simulink model "lead_acid_bat_eq_ckt_CC"  (R2025b)
settings: Solver=VariableStepAuto  StartTime=0.0  StopTime=200  RelTol=1e-3
libraries: fl_lib x16, nesl_utility x9, ee_lib x2
settings Model: Creator=huhry  LastModifiedBy=Hari
settings DebuggingCC: AlgebraicLoopMsg=none

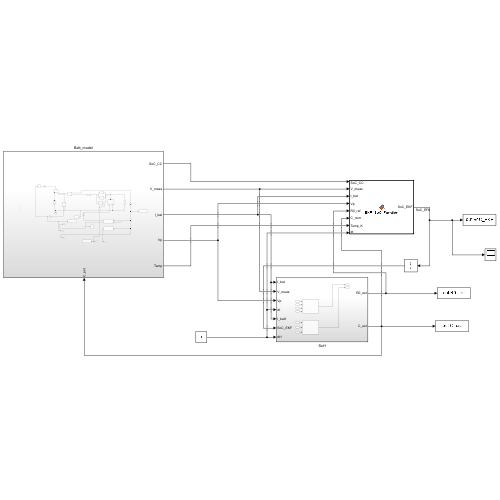
[thumbnail: Simulink's stored preview of the top-level diagram]
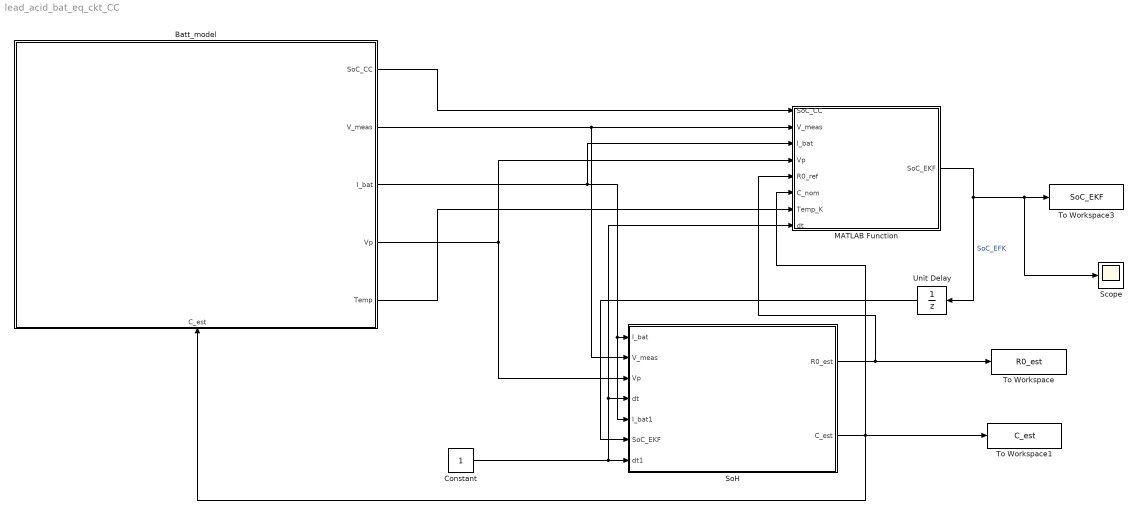
== system lead_acid_bat_eq_ckt_CC ==
  Batt_model : Subsystem
      settings: PortSchema="{\"entries\":[{\"content\":{\"sides\":[{\"content\":{},\"type\":\"ConnectorPlacement.EquallySpacedRectSide\",\"uuid\":\"49c69b95-09c6-49fd-b891-4f09856a00b3\"},{\"content\":{\"connectorIds\":[\"Out1\",\"Out2\",\"Out3\",\"Out4\",\"Out5\"],\"side\":\"RIGHT\"},\"type\":\"ConnectorPlacement.EquallySpacedRectSide\",\"uuid\":\"811e1f4c-4865-4a20-acff-08171fe05a53\"},{\"content\":{\"side\":\"TOP\"},\"type\":\"ConnectorPlacement.EquallySpacedRectSide\",\"uuid\":\"82a5ceef-4616-42bd-9951-d3b757a6a369\"},{\"content\":{\"connectorIds\":[\"In1\"],\"side\":\"BOTTOM\"},\"type\":\"ConnectorPlacement.EquallySpacedRectSide\",\"uuid\":\"0331ad85-3468-4588-880b-20861dbd2507\"}]},\"type\":\"ConnectorPlacement.EquallySpacedConnector\",\"uuid\":\"59096161-8cd8-4eb0-902d-7fdbb6e4005d\"}],\"packageUris\":[\"http://schema.mathworks.com/mf0/Connector/R2020b\"],\"version\":\"1.0\"}"
  Constant : Constant
  MATLAB Function : MATLAB Function  TreatAsAtomicUnit=on  SystemSampleTime=1
  Scope : Scope
      settings: ActiveDisplayYMinimum=-0.0893057108045884  ActiveDisplayYMaximum=1.1210339678671766
  SoH : Subsystem
  To Workspace : ToWorkspace  VariableName=R0_est  SaveFormat=Timeseries  SampleTime=-1
  To Workspace1 : ToWorkspace  VariableName=C_est  SaveFormat=Timeseries  SampleTime=-1
  To Workspace3 : ToWorkspace  VariableName=SoC_EKF  SaveFormat=Timeseries  SampleTime=-1
  Unit Delay : UnitDelay  InitialCondition=0.1  HasFrameUpgradeWarning=on
  wires:
  MATLAB Function/1(SoC_EKF) -> Unit Delay/1, Scope/1, To Workspace3/1  "SoC_EFK"
  Batt_model/1(SoC_CC) -> MATLAB Function/1(SoC_CC)
  Batt_model/2(V_meas) -> SoH/2(V_meas), MATLAB Function/2(V_meas)
  Batt_model/3(I_bat) -> SoH/5(I_bat1), SoH/1(I_bat), MATLAB Function/3(I_bat)
  Batt_model/4(Vp) -> SoH/3(Vp), MATLAB Function/4(Vp)
  Batt_model/5(Temp) -> MATLAB Function/7(Temp_K)
  SoH/1(R0_est) -> To Workspace/1, MATLAB Function/5(R0_ref)
  Constant/1 -> MATLAB Function/8(dt), SoH/4(dt), SoH/7(dt1)
  Unit Delay/1 -> SoH/6(SoC_EKF)
  SoH/2(C_est) -> Batt_model/1(C_est), To Workspace1/1, MATLAB Function/6(C_nom)

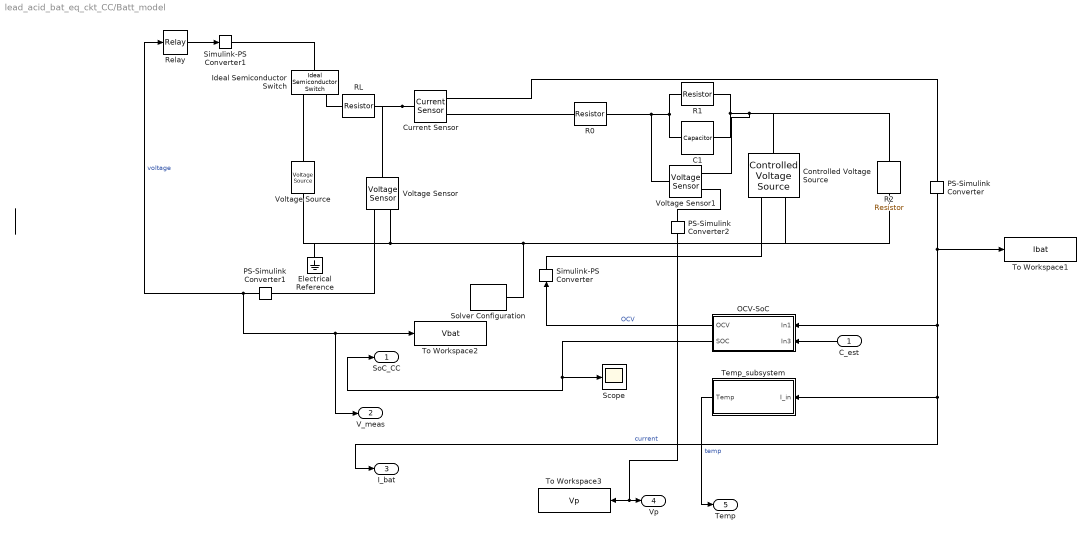
== system lead_acid_bat_eq_ckt_CC/Batt_model ==
  C_est : Inport
  C1 : fl_lib/Electrical/Electrical Elements/Capacitor  c=1000 F  r=1e-6 Ohm  g=0 1/Ohm  i_specify=off  i_priority=None  i=0 A  i_nominal_specify=off  i_nominal_value=1  i_nominal_unit=A  v_specify=off  v_priority=None  v=0 V  v_nominal_specify=off  v_nominal_value=1  v_nominal_unit=V  vc_specify=off  vc_priority=High  vc=0 V  vc_nominal_specify=off  vc_nominal_value=1  vc_nominal_unit=V
  Controlled Voltage Source : fl_lib/Electrical/Electrical Sources/Controlled Voltage Source
  Current Sensor : fl_lib/Electrical/Electrical Sensors/Current Sensor
  Electrical Reference : fl_lib/Electrical/Electrical Elements/Electrical Reference
  Ideal Semiconductor Switch : ee_lib/Semiconductors & Converters/Ideal Semiconductor Switch  port_option=ee.enum.controlport.ps  Ron=0.001 Ohm  Goff=1e-6 1/Ohm  Vth=0.5 V  diode_param=ee.enum.semiconductors.protectionDiode.external  diode_Vf=0.8 V  diode_Ron=0.001 Ohm  diode_Goff=1e-5 1/Ohm  diode_C=50e-9 F  diode_iRM=-235 A  diode_iF=300 A  diode_idot=-50 A/us  diode_trr_param=ee.enum.converters.diodetrr.trr_factor  diode_trr_factor=3  diode_trr=15 us  diode_Qrr=1500 s*uA
  OCV-SoC : Subsystem
  PS-Simulink Converter : nesl_utility/PS-Simulink Converter  PhysicalDomain=network_engine_domain  SubClassName=ps_output  LeftPortType=input  RightPortType=output  PseudoPeriodic=off  Frequencies=[]  VectorFormat=inherit  Unit=inherit  AffineConversion=off
  PS-Simulink Converter1 : nesl_utility/PS-Simulink Converter  PhysicalDomain=network_engine_domain  SubClassName=ps_output  LeftPortType=input  RightPortType=output  PseudoPeriodic=off  Frequencies=[]  VectorFormat=inherit  Unit=inherit  AffineConversion=off
  PS-Simulink Converter2 : nesl_utility/PS-Simulink Converter  PhysicalDomain=network_engine_domain  SubClassName=ps_output  LeftPortType=input  RightPortType=output  PseudoPeriodic=off  Frequencies=[]  VectorFormat=inherit  Unit=inherit  AffineConversion=off
  R0 : fl_lib/Electrical/Electrical Elements/Resistor  R=0.05 Ohm  i_specify=off  i_priority=None  i=0 A  i_nominal_specify=off  i_nominal_value=1  i_nominal_unit=A  v_specify=off  v_priority=None  v=0 V  v_nominal_specify=off  v_nominal_value=1  v_nominal_unit=V
  R1 : fl_lib/Electrical/Electrical Elements/Resistor  R=0.2 Ohm  i_specify=off  i_priority=None  i=0 A  i_nominal_specify=off  i_nominal_value=1  i_nominal_unit=A  v_specify=off  v_priority=None  v=0 V  v_nominal_specify=off  v_nominal_value=1  v_nominal_unit=V
  R2 : fl_lib/Electrical/Electrical Elements/Resistor  R=10000 Ohm  i_specify=off  i_priority=None  i=0 A  i_nominal_specify=off  i_nominal_value=1  i_nominal_unit=A  v_specify=off  v_priority=None  v=0 V  v_nominal_specify=off  v_nominal_value=1  v_nominal_unit=V
  RL : fl_lib/Electrical/Electrical Elements/Resistor  R=2 Ohm  i_specify=off  i_priority=None  i=0 A  i_nominal_specify=off  i_nominal_value=1  i_nominal_unit=A  v_specify=off  v_priority=None  v=0 V  v_nominal_specify=off  v_nominal_value=1  v_nominal_unit=V
  Relay : Relay  OnSwitchValue=14.4  OffSwitchValue=11  OnOutputValue=0  OffOutputValue=1
  Scope : Scope
      settings: ActiveDisplayYMinimum=-0.0090117486246958922  ActiveDisplayYMaximum=0.41517348204698179  DataLoggingVariableName=ScopeData2
  Simulink-PS Converter : nesl_utility/Simulink-PS Converter  PhysicalDomain=network_engine_domain  SubClassName=ps_input  LeftPortType=input  RightPortType=output  PseudoPeriodic=off  Frequencies=[]  NoiseDistribution=none  NoiseParameters=[]  Unit=1  AffineConversion=off  FilteringAndDerivatives=provide  SimscapeFilterOrder=1  InputFilterTimeConstant=0.001  UdotUserProvided=0
  Simulink-PS Converter1 : nesl_utility/Simulink-PS Converter  PhysicalDomain=network_engine_domain  SubClassName=ps_input  LeftPortType=input  RightPortType=output  PseudoPeriodic=off  Frequencies=[]  NoiseDistribution=none  NoiseParameters=[]  Unit=1  AffineConversion=off  FilteringAndDerivatives=provide  SimscapeFilterOrder=1  InputFilterTimeConstant=0.001  UdotUserProvided=0
  Solver Configuration : nesl_utility/Solver Configuration  PhysicalDomain=network_engine_domain  SubClassName=solver  LeftPortType=input  RightPortType=generic  Tones=[]  Harmonics=[]  SimulateNoise=off  Profile=off  UseLocalSampling=off  EnableSwitchedLinearOptims=on  FrequencyDomain=off  UseCCode=off  RelTol=0.001  AbsTol=0.001  MinStep=1e-09  ToWorkspace=off  RevertToSquareIcSolve=off  NumHomotopyIterations=100  PhasorMode=off  PhasorModeNumHarmonics=1  ConsistencySolver=NEWTON_XTOL_AFTER_FTOL  IndexReductionMethod=DerivativeReplacement  DoDC=off  ResidualTolerance=1e-09  ConsistencyTolSource=GLOBAL  ConsistencyAbsTol=0.001  ConsistencyRelTol=0.001  ConsistencyTolFactor=0.001  UseLocalSolver=off  LocalSolverChoice=NE_BACKWARD_EULER_ADVANCER  ResolveIndetEquations=on  FunctionEvalNumThread=1  LocalSolverSampleTime=0.001  DoFixedCost=off  MaxNonlinIter=3  MaxModeIter=2  ComputeImpulses=off  ImpulseIterations=2  LinearAlgebra=auto  LinearAlgebraNumThread=0  EquationFormulation=NE_TIME_EF  DelaysMemoryBudget=1024  AutomaticFiltering=on  FilteringTimeConstant=0.001  PartitionStorageMethod=AS_NEEDED  PartitionMemoryBudget=1024  PartitionMethod=ROBUST  MultibodyUseLocalSolver=off  MultibodyLocalSolverChoice=ODE1  MultibodyLocalSolverSampleTime=0.001
  Temp_subsystem : Subsystem
  To Workspace1 : ToWorkspace  VariableName=Ibat  SaveFormat=Timeseries  SampleTime=-1
  To Workspace2 : ToWorkspace  VariableName=Vbat  SaveFormat=Timeseries  SampleTime=-1
  To Workspace3 : ToWorkspace  VariableName=Vp  SaveFormat=Timeseries  SampleTime=-1
  Voltage Sensor : fl_lib/Electrical/Electrical Sensors/Voltage Sensor
  Voltage Sensor1 : fl_lib/Electrical/Electrical Sensors/Voltage Sensor
  Voltage Source : ee_lib/Sources/Voltage Source  dc_voltage=14 V  ac_voltage=0 V  ac_shift=0 rad  ac_frequency=60 Hz  noise_mode=ee.enum.sources.noise.Disabled  PSD=0 V^2/Hz  sample_time=1e-3 s  repeatability=ee.enum.sources.repeatability.NotRepeatable  user_seed=0  auto_seed=3499211588  i_specify=off  i_priority=None  i=0 A  i_nominal_specify=off  i_nominal_value=1  i_nominal_unit=A  v_specify=off  v_priority=None  v=0 V  v_nominal_specify=off  v_nominal_value=1  v_nominal_unit=V
  SoC_CC : Outport
  V_meas : Outport  Port=2
  I_bat : Outport  Port=3
  Vp : Outport  Port=4
  Temp : Outport  Port=5
  wires:
  OCV-SoC/1(OCV) -> Simulink-PS Converter/1  "OCV"
  PS-Simulink Converter1/1 -> V_meas/1, To Workspace2/1, Relay/1  "voltage"
  Relay/1 -> Simulink-PS Converter1/1
  PS-Simulink Converter2/1 -> Vp/1, To Workspace3/1
  PS-Simulink Converter/1 -> I_bat/1, Temp_subsystem/1(I_in), OCV-SoC/1(In1), To Workspace1/1  "current"
  Temp_subsystem/1(Temp) -> Temp/1  "temp"
  OCV-SoC/2(SOC) -> SoC_CC/1, Scope/1
  C_est/1 -> OCV-SoC/2(In3)
  connections:
  R1/RConn1 -- Voltage Sensor1/RConn2 -- Controlled Voltage Source/LConn1 -- R2/LConn1 -- C1/RConn1
  Solver Configuration/RConn1 -- Controlled Voltage Source/RConn2 -- R2/RConn1 -- Voltage Source/RConn1 -- Electrical Reference/LConn1 -- Voltage Sensor/RConn2
  R0/RConn1 -- Voltage Sensor1/LConn1 -- R1/LConn1 -- C1/LConn1
  Current Sensor/LConn1 -- Voltage Sensor/LConn1 -- RL/LConn1
  Ideal Semiconductor Switch/RConn1 -- RL/RConn1
  Current Sensor/RConn1 -- PS-Simulink Converter/LConn1
  Simulink-PS Converter1/RConn1 -- Ideal Semiconductor Switch/LConn1
  Voltage Sensor/RConn1 -- PS-Simulink Converter1/LConn1
  Simulink-PS Converter/RConn1 -- Controlled Voltage Source/RConn1
  PS-Simulink Converter2/LConn1 -- Voltage Sensor1/RConn1
  R0/LConn1 -- Current Sensor/RConn2
  ?
  Voltage Source/LConn1 -- Ideal Semiconductor Switch/RConn2

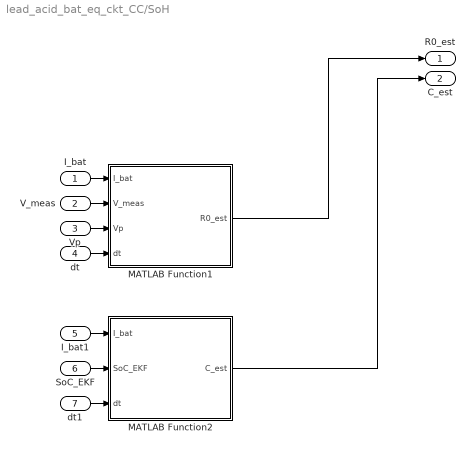
== system lead_acid_bat_eq_ckt_CC/SoH ==
  I_bat : Inport
  V_meas : Inport  Port=2
  Vp : Inport  Port=3
  dt : Inport  Port=4
  I_bat1 : Inport  Port=5
  SoC_EKF : Inport  Port=6
  dt1 : Inport  Port=7
  MATLAB Function1 : MATLAB Function  TreatAsAtomicUnit=on
  MATLAB Function2 : MATLAB Function  TreatAsAtomicUnit=on
  R0_est : Outport
  C_est : Outport  Port=2
  wires:
  dt/1 -> MATLAB Function1/4(dt)
  I_bat/1 -> MATLAB Function1/1(I_bat)
  MATLAB Function1/1(R0_est) -> R0_est/1
  V_meas/1 -> MATLAB Function1/2(V_meas)
  MATLAB Function2/1(C_est) -> C_est/1
  I_bat1/1 -> MATLAB Function2/1(I_bat)
  SoC_EKF/1 -> MATLAB Function2/2(SoC_EKF)
  Vp/1 -> MATLAB Function1/3(Vp)
  dt1/1 -> MATLAB Function2/3(dt)

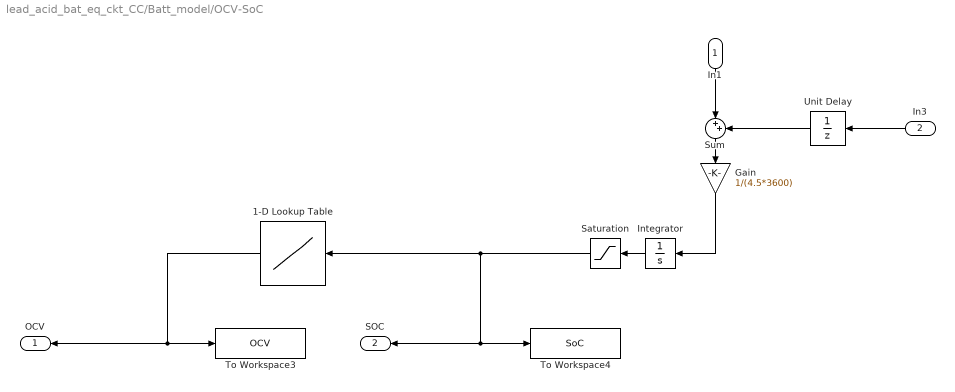
== system lead_acid_bat_eq_ckt_CC/Batt_model/OCV-SoC ==
  In1 : Inport
  In3 : Inport  Port=2
  1-D Lookup Table : Lookup_n-D  NumberOfTableDimensions=1  BreakpointsForDimension1=[0, 0.1, 0.2, 0.3, 0.4, 0.5, 0.6, 0.7, 0.8, 0.9, 1]  Table=[11.0, 11.5, 11.8, 12.0, 12.2, 12.4, 12.6, 12.8, 13.0, 13.5, 13.8]  ExtrapMethod=Clip  InternalRulePriority=Speed  RndMeth=Simplest
  Gain : Gain  Gain=1/(4.5*3600)
  Integrator : Integrator  InitialCondition=0.1
  Saturation : Saturate  UpperLimit=1  LowerLimit=0
  Sum : Sum  Inputs=|++
  To Workspace3 : ToWorkspace  VariableName=OCV  SaveFormat=Timeseries  SampleTime=-1
  To Workspace4 : ToWorkspace  VariableName=SoC  SaveFormat=Timeseries  SampleTime=-1
  Unit Delay : UnitDelay  HasFrameUpgradeWarning=on
  OCV : Outport
  SOC : Outport  Port=2
  wires:
  Gain/1 -> Integrator/1
  1-D Lookup Table/1 -> To Workspace3/1, OCV/1
  Integrator/1 -> Saturation/1
  Saturation/1 -> SOC/1, To Workspace4/1, 1-D Lookup Table/1
  In3/1 -> Unit Delay/1
  Sum/1 -> Gain/1
  In1/1 -> Sum/1
  Unit Delay/1 -> Sum/2

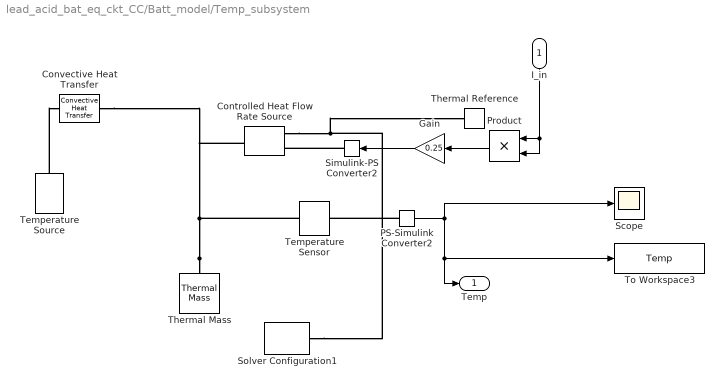
== system lead_acid_bat_eq_ckt_CC/Batt_model/Temp_subsystem ==
  I_in : Inport
  Controlled Heat Flow Rate Source : fl_lib/Thermal/Thermal Sources/Controlled Heat Flow Rate Source
  Convective Heat Transfer : fl_lib/Thermal/Thermal Elements/Convective Heat Transfer  thermal_type=foundation.enum.constant_variable.constant  area=1e-4 m^2  heat_tr_coeff=20 W/(K*m^2)  min_heat_tr_coeff=1e-3 W/(K*m^2)  T_specify=off  T_priority=None  T=0 K  T_nominal_specify=off  T_nominal_value=1  T_nominal_unit=K  Q_specify=off  Q_priority=None  Q=0 W  Q_nominal_specify=off  Q_nominal_value=1  Q_nominal_unit=W
  Gain : Gain  Gain=0.25
  PS-Simulink Converter2 : nesl_utility/PS-Simulink Converter  PhysicalDomain=network_engine_domain  SubClassName=ps_output  LeftPortType=input  RightPortType=output  PseudoPeriodic=off  Frequencies=[]  VectorFormat=inherit  Unit=inherit  AffineConversion=off
  Product : Product
  Scope : Scope
      settings: ActiveDisplayYMinimum=-1  ActiveDisplayYMaximum=1
  Simulink-PS Converter2 : nesl_utility/Simulink-PS Converter  PhysicalDomain=network_engine_domain  SubClassName=ps_input  LeftPortType=input  RightPortType=output  PseudoPeriodic=off  Frequencies=[]  NoiseDistribution=none  NoiseParameters=[]  Unit=1  AffineConversion=off  FilteringAndDerivatives=provide  SimscapeFilterOrder=1  InputFilterTimeConstant=0.001  UdotUserProvided=0
  Solver Configuration1 : nesl_utility/Solver Configuration  PhysicalDomain=network_engine_domain  SubClassName=solver  LeftPortType=input  RightPortType=generic  Tones=[]  Harmonics=[]  SimulateNoise=off  Profile=off  UseLocalSampling=off  EnableSwitchedLinearOptims=on  FrequencyDomain=off  UseCCode=off  RelTol=0.001  AbsTol=0.001  MinStep=1e-09  ToWorkspace=off  RevertToSquareIcSolve=off  NumHomotopyIterations=100  PhasorMode=off  PhasorModeNumHarmonics=1  ConsistencySolver=NEWTON_XTOL_AFTER_FTOL  IndexReductionMethod=DerivativeReplacement  DoDC=off  ResidualTolerance=1e-09  ConsistencyTolSource=GLOBAL  ConsistencyAbsTol=0.001  ConsistencyRelTol=0.001  ConsistencyTolFactor=0.001  UseLocalSolver=off  LocalSolverChoice=NE_BACKWARD_EULER_ADVANCER  ResolveIndetEquations=on  FunctionEvalNumThread=1  LocalSolverSampleTime=0.001  DoFixedCost=off  MaxNonlinIter=3  MaxModeIter=2  ComputeImpulses=off  ImpulseIterations=2  LinearAlgebra=auto  LinearAlgebraNumThread=0  EquationFormulation=NE_TIME_EF  DelaysMemoryBudget=1024  AutomaticFiltering=on  FilteringTimeConstant=0.001  PartitionStorageMethod=AS_NEEDED  PartitionMemoryBudget=1024  PartitionMethod=ROBUST  MultibodyUseLocalSolver=off  MultibodyLocalSolverChoice=ODE1  MultibodyLocalSolverSampleTime=0.001
  Temperature Sensor : fl_lib/Thermal/Thermal Sensors/Temperature Sensor  temperature_measure=foundation.enum.MeasurementReference.absolute
      settings: InternalSimscapePortConfiguration="{\"Bottom\":[],\"Left\":[{\"id\":\"A\",\"label\":\"A\",\"type\":\"foundation.thermal.thermal\"}],\"Right\":[{\"id\":\"T\",\"label\":\"T\",\"type\":\"output\"}],\"Top\":[]}"
  Temperature Source : fl_lib/Thermal/Thermal Sources/Temperature Source  temperature=298.15 K
  Thermal Mass : fl_lib/Thermal/Thermal Elements/Thermal Mass  mass_type=foundation.enum.constant_variable.constant  mass=1 kg  sp_heat=900 J/(K*kg)  mass_min=1e-6 kg  num_ports=foundation.enum.numPorts2.one  m_specify=off  m_priority=High  m=1 kg  m_nominal_specify=off  m_nominal_value=1  m_nominal_unit=kg  T_specify=on  T_priority=High  T=298.15 K  T_nominal_specify=off  T_nominal_value=1  T_nominal_unit=K  Q_specify=off  Q_priority=None  Q=0 W  Q_nominal_specify=off  Q_nominal_value=1  Q_nominal_unit=W
  Thermal Reference : fl_lib/Thermal/Thermal Elements/Thermal Reference
  To Workspace3 : ToWorkspace  VariableName=Temp  SaveFormat=Timeseries  SampleTime=-1
  Temp : Outport
  wires:
  Gain/1 -> Simulink-PS Converter2/1
  I_in/1 -> Product/2, Product/1
  PS-Simulink Converter2/1 -> Temp/1, To Workspace3/1, Scope/1
  Product/1 -> Gain/1
  connections:
  Thermal Mass/LConn1 -- Controlled Heat Flow Rate Source/LConn1 -- Convective Heat Transfer/LConn1 -- Temperature Sensor/LConn1
  Controlled Heat Flow Rate Source/RConn2 -- Solver Configuration1/RConn1 -- Thermal Reference/LConn1
  Temperature Source/LConn1 -- Convective Heat Transfer/RConn1
  Simulink-PS Converter2/RConn1 -- Controlled Heat Flow Rate Source/RConn1
  PS-Simulink Converter2/LConn1 -- Temperature Sensor/RConn1

== matlab function lead_acid_bat_eq_ckt_CC/SoH/MATLAB Function1 ==
  settings: updateMethod=DISCRETE
  data: I_bat input; R0_est output; V_meas input; Vp input; dt input
function R0_est = SoH_R0(I_bat, V_meas, Vp, dt)
%#codegen
persistent R0 V_prev I_prev

if isempty(R0)
    R0 = 0.02;   % initial guess (ohms)
    V_prev = V_meas;
    I_prev = I_bat;
end

% Detect current step
dI = I_bat - I_prev;
dV = V_meas - V_prev;

I_thresh = 1.0;

if abs(dI) > I_thresh
    R0_new = abs(dV / dI);
    % Slow update (low-pass)
    alpha = 0.01;
    R0 = (1 - alpha)*R0 + alpha*R0_new;
end

% Store previous values
V_prev = V_meas;
I_prev = I_bat;

R0_est = max(R0, 0.005);  % safety clamp
end

== matlab function lead_acid_bat_eq_ckt_CC/MATLAB Function ==
  settings: updateMethod=DISCRETE
  data: SoC_CC input; SoC_EKF output; V_meas input; I_bat input; Vp input; R0_ref input; C_nom input; Temp_K input; dt input
function SoC_EKF = EKF_SoC_Function( ...
    SoC_CC, V_meas, I_bat, Vp, ...
    R0_ref, C_nom, Temp_K, dt)
%#codegen
% Single-State EKF for SoC (1-RC, Temp-aware, SoH-ready)

%% ================= Persistent States =================
persistent x_hat P
if isempty(x_hat)
    x_hat = SoC_CC;   % Initialize from CC
    P     = 1e-3;
end

%% ================= Tuning =================
R = 1e-2;    % Voltage noise
Q = 1e-6;    % Process noise
Delta = 1e-3;

%% ================= Temperature Model =================
T_ref   = 298.15;
alpha_T = -0.003;

R0_eff = R0_ref * (1 + alpha_T * (Temp_K - T_ref));
R0_eff = max(R0_eff, 0.2 * R0_ref);

%% ================= OCV LUT =================
persistent soc_bp ocv_table
if isempty(soc_bp)
    soc_bp = 0:0.1:1.0;
    ocv_table = [11.6 11.9 12.1 12.3 12.5 ...
                 12.7 12.9 13.1 13.3 13.6 13.8];
end

%% ================= PREDICTION =================
% EKF physical prediction using capacity (SoH)
x_pred = x_hat + (I_bat * dt) / C_nom;

% Clamp
x_pred = min(max(x_pred, 0), 1);

% Covariance prediction
P_pred = P + Q;

%% ================= Measurement Model =================
OCV = interp1(soc_bp, ocv_table, x_pred, 'linear', 'extrap');

SoC_p = min(max(x_pred + Delta, 0), 1);
SoC_m = min(max(x_pred - Delta, 0), 1);

OCV_p = interp1(soc_bp, ocv_table, SoC_p, 'linear', 'extrap');
OCV_m = interp1(soc_bp, ocv_table, SoC_m, 'linear', 'extrap');

H = (OCV_p - OCV_m) / (2 * Delta);

V_pred = OCV - Vp - I_bat * R0_eff;

%% ================= UPDATE =================
residual = V_meas - V_pred;

S = H * P_pred * H + R;
K = (P_pred * H) / S;

x_hat = x_pred + K * residual;
x_hat = min(max(x_hat, 0), 1);

P = (1 - K * H) * P_pred;

SoC_EKF = x_hat;

end

== matlab function lead_acid_bat_eq_ckt_CC/SoH/MATLAB Function2 ==
  settings: updateMethod=DISCRETE
  data: I_bat input; C_est output; SoC_EKF input; dt input
function C_est = SoH_Capacity(I_bat, SoC_EKF, dt)
%#codegen
% Slow SoH estimator for battery capacity (Coulombs)

%% ================= Persistent States =================
persistent Q_acc SoC_start C

if isempty(Q_acc)
    Q_acc     = 0;                 % Accumulated charge (Coulombs)
    SoC_start = SoC_EKF;            % SoC at start of window
    C         = 20 * 3600;          % INITIAL capacity (20Ah -> Coulombs)
end

%% ================= Charge Accumulation =================
Q_acc = Q_acc + I_bat * dt;         % I in A, dt in s → Coulombs

%% ================= SoC Change =================
delta_SoC = SoC_EKF - SoC_start;

%% ================= Capacity Update Condition =================
% Update only when enough SoC change has occurred
if abs(delta_SoC) > 0.05            % 5% SoC window

    C_new = abs(Q_acc / delta_SoC); % Capacity estimate (Coulombs)

    % Very slow learning (SoH must be boring)
    beta = 0.005;
    C = (1 - beta)*C + beta*C_new;

    % Reset accumulation window
    Q_acc     = 0;
    SoC_start = SoC_EKF;
end

%% ================= Safety Clamp =================
C_nom_initial = 20 * 3600;           % Nominal capacity (Coulombs)
C_est = max(C, 0.5 * C_nom_initial); % Prevent collapse

end
